simulink model "EV3robot_SIMmodelV2017b"  (R2019b)
settings: Solver=VariableStepAuto  StartTime=0.0  StopTime=60  RelTol=1e-3
values from neighbouring files (symbols this model uses):
  Kc = 5    [EV3robot_model_param.m]
  Km = 14.72    [EV3robot_model_param.m]
  SqWaveFreq = 1/6    (= 0.166666666667)    [EV3robot_model_param.m]
  ThDotRef = 360    [EV3robot_model_param.m]
  Tm = 0.028    [EV3robot_model_param.m]
  Ts = 0.005    [EV3robot_model_param.m]
  Vm = 30    [EV3robot_model_param.m]
undefined symbols (not defined in the file or in its folder): COLden, COLnum, DiscIntNeverNeededParam, qdotwmr
libraries: simulink x1
settings Model: Creator=mwcant  LastModifiedBy=linesLK
settings DebuggingCC: ArithmeticOperatorsInVariantConditions=warning
settings SFSimCC: CustomCodeUndefinedFunction=UseInterfaceOnly

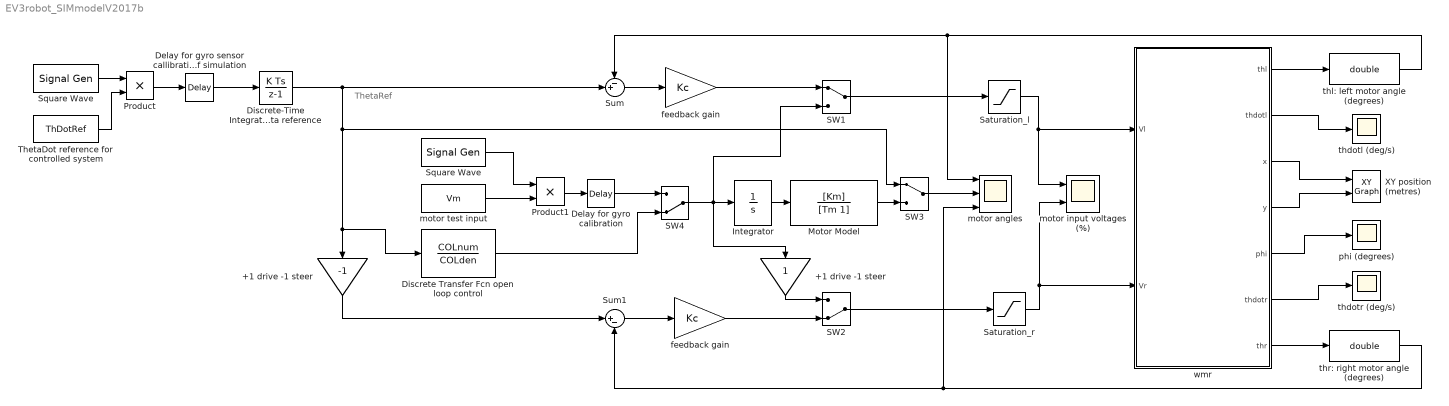
== system EV3robot_SIMmodelV2017b ==
  note: ThetaRef
  +1 drive -1 steer : Gain  Gain=-1
  "+1 drive -1 steer " : Gain
  Delay for gyro calibration : TransportDelay  DelayTime=2  FixedBuffer=on
  "Delay for gyro sensor callibration at start of simulation " : TransportDelay  DelayTime=2  FixedBuffer=on
  Discrete Transfer Fcn open loop control : DiscreteTransferFcn  Numerator=COLnum  Denominator=COLden  SampleTime=Ts
  Discrete-Time Integrator to convert ThetaDot reference to a Theta reference : DiscreteIntegrator  SampleTime=Ts  ICPrevOutput=DiscIntNeverNeededParam  ICPrevScaledInput=DiscIntNeverNeededParam
  Integrator : Integrator
  Motor Model : TransferFcn  Numerator=[Km]  Denominator=[Tm 1]
  Product : Product
  Product1 : Product
  SW1 : ManualSwitch
  SW2 : ManualSwitch  CurrentSetting=0
  SW3 : ManualSwitch
  SW4 : ManualSwitch  CurrentSetting=0
  Saturation_l : Saturate  UpperLimit=100  LowerLimit=-100
  "Saturation_r " : Saturate  UpperLimit=100  LowerLimit=-100
  Square Wave : SignalGenerator  WaveForm=square  Frequency=SqWaveFreq
  "Square Wave " : SignalGenerator  WaveForm=square  Frequency=SqWaveFreq
  Sum : Sum  Inputs=-+|
  Sum1 : Sum  Inputs=|+-
  ThetaDot reference for controlled system : Constant  Value=ThDotRef
  XY position (metres) : simulink/Sinks/XY Graph  xmin=-0.5  xmax=0.5  ymin=-0.1  ymax=0.1  st=-1
  feedback gain : Gain  Gain=Kc
  "feedback gain " : Gain  Gain=Kc
  motor angles : Scope  NumInputPorts=3
  "motor input voltages (%) " : Scope  NumInputPorts=2
  motor test input : Constant  Value=Vm
  phi (degrees) : Scope
  thdotl (deg/s) : Scope
  thdotr (deg/s) : Scope
  thl: left motor angle (degrees) : DataTypeConversion  OutDataTypeStr=double
  thr: right motor angle (degrees) : DataTypeConversion  OutDataTypeStr=double
  "wmr " : Subsystem
  wires:
  +1 drive -1 steer/1 -> Sum1/1
  "wmr "/6(thdotr) -> thdotr (deg/s)/1
  Sum/1 -> feedback gain/1
  feedback gain/1 -> SW1/1
  "Square Wave "/1 -> Product1/1
  "+1 drive -1 steer "/1 -> SW2/1
  Sum1/1 -> "feedback gain "/1
  Discrete-Time Integrator to convert ThetaDot reference to a Theta reference/1 -> +1 drive -1 steer/1, Discrete Transfer Fcn open loop control/1, SW3/1, Sum/2
  "wmr "/2(thdotl) -> thdotl (deg/s)/1
  Motor Model/1 -> SW3/2
  thl: left motor angle (degrees)/1 -> motor angles/1, Sum/1
  "wmr "/1(thl) -> thl: left motor angle (degrees)/1
  SW2/1 -> "Saturation_r "/1
  Integrator/1 -> Motor Model/1
  "Delay for gyro sensor callibration at start of simulation "/1 -> Discrete-Time Integrator to convert ThetaDot reference to a Theta reference/1
  "wmr "/7(thr) -> thr: right motor angle (degrees)/1
  SW4/1 -> Integrator/1, SW1/2, "+1 drive -1 steer "/1
  Product1/1 -> Delay for gyro calibration/1
  "feedback gain "/1 -> SW2/2
  "wmr "/5(phi) -> phi (degrees)/1
  Product/1 -> "Delay for gyro sensor callibration at start of simulation "/1
  ThetaDot reference for controlled system/1 -> Product/2
  Discrete Transfer Fcn open loop control/1 -> SW4/2
  "wmr "/3(x) -> XY position (metres)/1
  Square Wave/1 -> Product/1
  SW1/1 -> Saturation_l/1
  "wmr "/4(y) -> XY position (metres)/2
  motor test input/1 -> Product1/2
  thr: right motor angle (degrees)/1 -> motor angles/3, Sum1/2
  Delay for gyro calibration/1 -> SW4/1
  SW3/1 -> motor angles/2
  Saturation_l/1 -> "motor input voltages (%) "/1, "wmr "/1(Vl)
  "Saturation_r "/1 -> "motor input voltages (%) "/2, "wmr "/2(Vr)

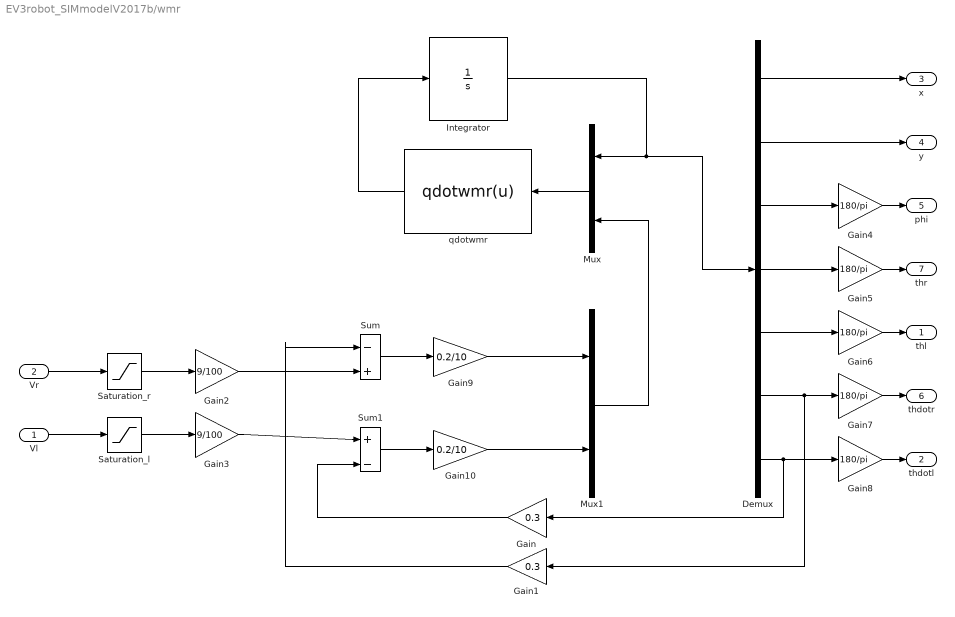
== system EV3robot_SIMmodelV2017b/wmr  ==
  Vl : Inport
  Vr : Inport  Port=2
  Demux : Demux  Outputs=7
  Gain : Gain  Gain=0.3
  Gain1 : Gain  Gain=0.3
  Gain10 : Gain  Gain=0.2/10
  Gain2 : Gain  Gain=9/100
  Gain3 : Gain  Gain=9/100
  Gain{4..8} (5 alike) : Gain  Gain=180/pi
  Gain9 : Gain  Gain=0.2/10
  Integrator : Integrator  InitialCondition=[0; 0; 0; 0; 0; 0; 0]
  Mux : Mux  Inputs=2
  Mux1 : Mux  Inputs=2
  Saturation_l : Saturate  UpperLimit=100  LowerLimit=-100
  "Saturation_r " : Saturate  UpperLimit=100  LowerLimit=-100
  Sum : Sum  Inputs=-|+
  Sum1 : Sum  Inputs=+|-
  qdotwmr : MATLABFcn  MATLABFcn=qdotwmr(u)
  thl : Outport
  thdotl : Outport  Port=2
  x : Outport  Port=3
  y : Outport  Port=4
  phi : Outport  Port=5
  thdotr : Outport  Port=6
  thr : Outport  Port=7
  wires:
  Vr/1 -> "Saturation_r "/1
  Vl/1 -> Saturation_l/1
  Demux/1 -> x/1
  Sum/1 -> Gain9/1
  Gain9/1 -> Mux1/1
  Gain10/1 -> Mux1/2
  Demux/6 -> Gain7/1, Gain1/1
  Mux/1 -> qdotwmr/1
  Integrator/1 -> Demux/1, Mux/1
  Demux/7 -> Gain8/1, Gain/1
  Gain1/1 -> Sum/1
  qdotwmr/1 -> Integrator/1
  Mux1/1 -> Mux/2
  Sum1/1 -> Gain10/1
  Demux/2 -> y/1
  Gain/1 -> Sum1/2
  "Saturation_r "/1 -> Gain2/1
  Saturation_l/1 -> Gain3/1
  Gain2/1 -> Sum/2
  Gain3/1 -> Sum1/1
  Demux/3 -> Gain4/1
  Gain4/1 -> phi/1
  Gain5/1 -> thr/1
  Demux/4 -> Gain5/1
  Gain6/1 -> thl/1
  Demux/5 -> Gain6/1
  Gain7/1 -> thdotr/1
  Gain8/1 -> thdotl/1
